simulink model "frequency_band_state_controller_sim"  (R2020b)
settings: Solver=VariableStepAuto  StartTime=0.0  StopTime=stop_time  RelTol=1e-3
InitFcn:
  | frequency_band_state_controller_sim_init
StopFcn:
  | frequency_band_state_controller_sim_stop
undefined symbols (not defined in the file or in its folder): fs
libraries: dspsrcs4 x1
settings Model: Creator=t96f346  LastModifiedBy=t96f346

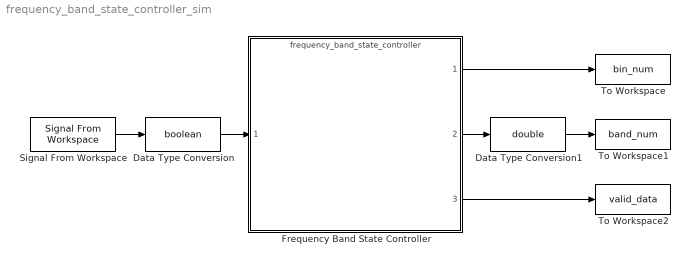
== system frequency_band_state_controller_sim ==
  Data Type Conversion : DataTypeConversion  OutDataTypeStr=boolean
  Data Type Conversion1 : DataTypeConversion  OutDataTypeStr=double
  Frequency Band State Controller : ModelReference  ModelNameDialog=frequency_band_state_controller  SimulationMode=Normal  ModelReferenceVersion=2.30
  Signal From Workspace : dspsrcs4/Signal From Workspace  X=valid_data  Ts=1/fs  nsamps=1  OutputAfterFinalValue=Setting to zero  ignoreOrWarnInputAndFrameLengths=off  OutputFrames=off
  To Workspace : ToWorkspace  VariableName=bin_num  SampleTime=-1
      settings: Save2DSignal=2-D array (concatenate along first dimension)
  To Workspace1 : ToWorkspace  VariableName=band_num  SampleTime=-1
      settings: Save2DSignal=2-D array (concatenate along first dimension)
  To Workspace2 : ToWorkspace  VariableName=valid_data  SampleTime=-1
      settings: Save2DSignal=2-D array (concatenate along first dimension)
  wires:
  Signal From Workspace/1 -> Data Type Conversion/1
  Frequency Band State Controller/1 -> To Workspace/1
  Frequency Band State Controller/2 -> Data Type Conversion1/1
  Frequency Band State Controller/3 -> To Workspace2/1
  Data Type Conversion/1 -> Frequency Band State Controller/1
  Data Type Conversion1/1 -> To Workspace1/1
